simulink model "test_topo"  (R2023b)
settings: Solver=FixedStepAuto  StartTime=0  StopTime=0.1e-3  FixedStep=1e-9  RelTol=1e-3
values from neighbouring files (symbols this model uses):
  C = 34e-6    (= 3.4e-05)    [code_lsandtrain.m]
  It = 2310    [code_lsandtrain.m]
  L = 3.5e-6    (= 3.5e-06)    [code_lsandtrain.m]
  Lc = Lc*2    (= 8e-07)    [code_lsandtrain.m]
  Ld = 2.5e-7    (= 2.5e-07)    [code_lsandtrain.m]
  Lr = 3e-7    (= 3e-07)    [code_lsandtrain.m]
  R = 0.65    [code_lsandtrain.m]
  Ud = 2500    [code_lsandtrain.m]
undefined symbols (not defined in the file or in its folder): Udc
libraries: spsSeriesRLCBranchLib x47, spsVoltageMeasurementLib x38, spsDiodeLib x18, spsControlledCurrentSourceLib x9, spsCurrentMeasurementLib x9, spsDCVoltageSourceLib x9, spsIGBTDiodeLib x9, sps_lib x1
settings Model: Creator=Jhchen  LastModifiedBy=Jhchen
settings DataIOCC: ReturnWorkspaceOutputs=off

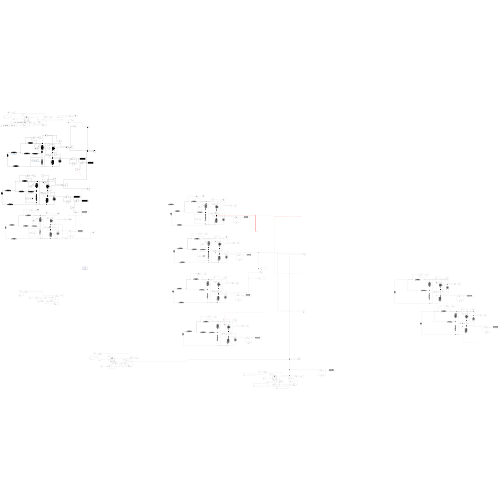
[thumbnail: Simulink's stored preview of the top-level diagram]
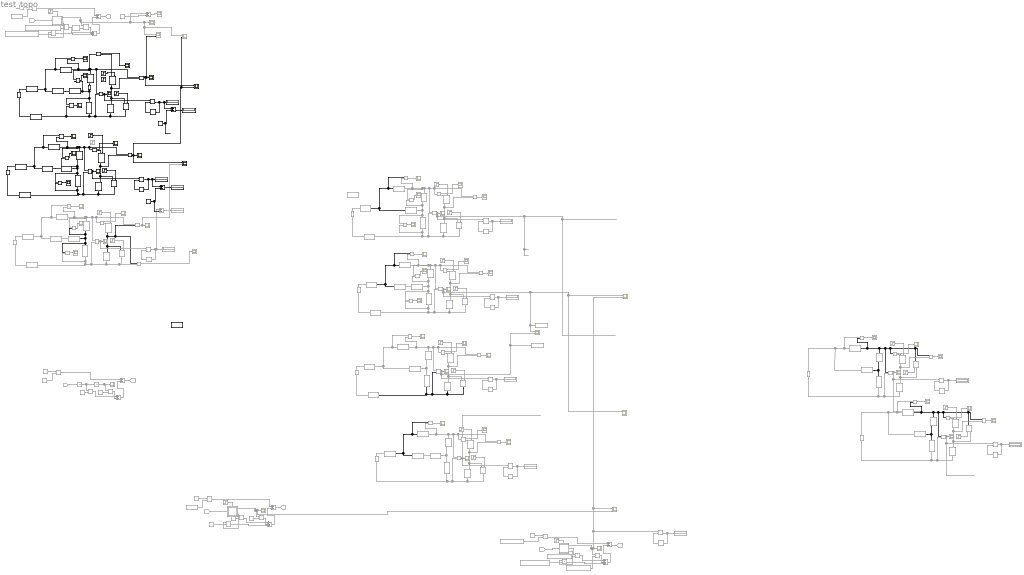
== system test_topo ==
  Add : Sum  Commented=on
  Add{1,3,5,7,10..11} (6 alike) : Sum  Commented=on  Inputs=+-
  Add2 : Sum  Commented=on  Inputs=+++
  Add4 : Sum  Commented=on  Inputs=+++
  Add6 : Sum  Inputs=+-
  Add8 : Sum  Inputs=+-
  Add9 : Sum  Commented=on  Inputs=+++
  Constant : Constant  Commented=on  Value=2400
  Constant1 : Constant  Commented=on  Value=L*C
  Constant10 : Constant  Commented=on  Value=R/(L*Lr*C+L*Lc*C+Lc*Lr*C)
  Constant11 : Constant  Commented=on  Value=R/(L*Lr*C+L*Lc*C+Lc*Lr*C)
  Constant12 : Constant  Commented=on  Value=(L+Lr)/(L*Lr*C+L*Lc*C+Lc*Lr*C)
  Constant13 : Constant  Commented=on  Value=(L*R*C+Lc*C*R)/(L*Lr*C+L*Lc*C+Lc*Lr*C)
  Constant14 : Constant  Value=Ud
  Constant15 : Constant  Value=Ud
  Constant16 : Constant  Commented=on  Value=Ud
  Constant17 : Constant  Commented=on  Value=(C*(L*Lc+Lc*Ld+Lc*Lr+Lr*L+Lr*Ld))/R
  Constant18 : Constant  Commented=on  Value=C*(L*Lc+Lc*Ld+Lc*Lr+Lr*L+Lr*Ld)/R
  Constant19 : Constant  Commented=on  Value=C*(L*Lc+Lc*Ld+Lc*Lr+Lr*L+Lr*Ld)/((L+Ld+Lr))
  Constant2 : Constant  Commented=on  Value=L*C
  Constant20 : Constant  Commented=on  Value=C*(L*Lc+Lc*Ld+Lc*Lr+Lr*L+Lr*Ld)/(C*R*(Lc+L+Ld))
  Constant21 : Constant  Commented=on  Value=Ud
  Constant3 : Constant  Commented=on  Value=R*C
  Constant4 : Constant  Commented=on  Value=Udc
  Constant5 : Constant  Commented=on  Value=L*C*Lc/R
  Constant6 : Constant  Commented=on  Value=L*C*Lc/R
  Constant7 : Constant  Commented=on  Value=Lc*C
  Constant8 : Constant  Commented=on  Value=L*Lc/R/(Lc+L)
  Constant9 : Constant  Commented=on  Value=Udc
  Controlled Current Source{1..7} (7 alike) : spsControlledCurrentSourceLib/Controlled Current Source  Commented=on  Initialize=on  Source_Type=AC  Amplitude=0  Phase=0  Frequency=0  Measurements=None
  Controlled Current Source8 : spsControlledCurrentSourceLib/Controlled Current Source  Initialize=on  Source_Type=AC  Amplitude=0  Phase=0  Frequency=0  Measurements=None
  Controlled Current Source9 : spsControlledCurrentSourceLib/Controlled Current Source  Initialize=on  Source_Type=AC  Amplitude=0  Phase=0  Frequency=0  Measurements=None
  Current Measurement{1..7} (7 alike) : spsCurrentMeasurementLib/Current Measurement  Commented=on  PhasorSimulation=off  OutputType=Complex  PSBequivalent=0
  Current Measurement8 : spsCurrentMeasurementLib/Current Measurement  PhasorSimulation=off  OutputType=Complex  PSBequivalent=0
  Current Measurement9 : spsCurrentMeasurementLib/Current Measurement  PhasorSimulation=off  OutputType=Complex  PSBequivalent=0
  DC Voltage Source1 : spsDCVoltageSourceLib/DC Voltage Source  Commented=on  Amplitude=Udc  Measurements=None
  DC Voltage Source2 : spsDCVoltageSourceLib/DC Voltage Source  Commented=on  Amplitude=2400  Measurements=None
  DC Voltage Source3 : spsDCVoltageSourceLib/DC Voltage Source  Commented=on  Amplitude=2400  Measurements=None
  DC Voltage Source4 : spsDCVoltageSourceLib/DC Voltage Source  Commented=on  Amplitude=2400  Measurements=None
  DC Voltage Source5 : spsDCVoltageSourceLib/DC Voltage Source  Commented=on  Amplitude=Udc  Measurements=None
  DC Voltage Source6 : spsDCVoltageSourceLib/DC Voltage Source  Commented=on  Amplitude=2500  Measurements=None
  DC Voltage Source7 : spsDCVoltageSourceLib/DC Voltage Source  Commented=on  Amplitude=Ud  Measurements=None
  DC Voltage Source8 : spsDCVoltageSourceLib/DC Voltage Source  Amplitude=Ud  Measurements=None
  DC Voltage Source9 : spsDCVoltageSourceLib/DC Voltage Source  Amplitude=Ud  Measurements=None
  Delay{1..8} (8 alike) : Delay  Commented=on  DelayLength=1
  Delay10 : Delay  DelayLength=1
  Delay9 : Delay  DelayLength=1
  Diode{1..14} (14 alike) : spsDiodeLib/Diode  Commented=on  Ron=0.001  Lon=0  Vf=0.8  IC=0  UseSnubber=0  Rs=500  Cs=250e-9  Measurements=on
  Diode{15..18} (4 alike) : spsDiodeLib/Diode  Ron=0.001  Lon=0  Vf=0.8  IC=0  UseSnubber=0  Rs=500  Cs=250e-9  Measurements=on
  Display{1..8,11} (9 alike) : Display  Commented=on
  Display{9..10,12..13} (4 alike) : Display
  Divide{,1..6,11..14} (11 alike) : Product  Commented=on  Inputs=*/
  Divide{7..10} (4 alike) : Product  Commented=on  Inputs=**
  From : From  Commented=on  GotoTag=vc2
  From1 : From  Commented=on  GotoTag=vc3
  From2 : From  Commented=on  GotoTag=vc4
  From3 : From  Commented=on  GotoTag=vc3
  Goto : Goto  Commented=on  GotoTag=vc2
  Goto1 : Goto  Commented=on  GotoTag=vc3
  Goto2 : Goto  Commented=on  GotoTag=vc4
  Goto3 : Goto  Commented=on  GotoTag=vc3
  IGBT/Diode{1..7} (7 alike) : spsIGBTDiodeLib/IGBT//Diode  Commented=on  Ron=0.39e-3  Rs=1e5  Cs=inf  Measurements=on
  IGBT/Diode8 : spsIGBTDiodeLib/IGBT//Diode  Ron=0.39e-3  Rs=1e5  Cs=inf  Measurements=on
  IGBT/Diode9 : spsIGBTDiodeLib/IGBT//Diode  Ron=0.39e-3  Rs=1e5  Cs=inf  Measurements=on
  Integrator1 : Integrator  Commented=on  InitialCondition=2400
  Integrator3 : Integrator  Commented=on  InitialCondition=1750/C
  Max{1..8} (8 alike) : MinMax  Commented=on  Function=max  Inputs=2
  Max10 : MinMax  Function=max  Inputs=2
  Max9 : MinMax  Function=max  Inputs=2
  Scope : Scope  NumInputPorts=2
  Scope{1..3,5..11,13..24,26..28,30..41,48,56,59} (40 alike) : Scope  Commented=on
  Scope12 : Scope  Commented=on  NumInputPorts=4
  Scope25 : Scope  Commented=on  NumInputPorts=3
  Scope{4,29,57..58} (4 alike) : Scope  Commented=on  NumInputPorts=2
  Scope{42..47,50..55} (12 alike) : Scope
  Scope49 : Scope  NumInputPorts=2
  Series RLC Branch{1,16,21,27} (4 alike) : spsSeriesRLCBranchLib/Series RLC Branch  Commented=on  LConnTagsString=__new0  RConnTagsString=__new0  BranchType=L  Resistance=0.00001  Inductance=L  SetiL0=off  InitialCurrent=4000  Capacitance=1e-6  Setx0=off  InitialVoltage=0  Measurements=None
  Series RLC Branch10 : spsSeriesRLCBranchLib/Series RLC Branch  Commented=on  LConnTagsString=__new0  RConnTagsString=__new0  BranchType=L  Resistance=1  Inductance=L  SetiL0=off  InitialCurrent=0  Capacitance=1e-6  Setx0=off  InitialVoltage=0  Measurements=None
  Series RLC Branch{4..6,11,24,34} (6 alike) : spsSeriesRLCBranchLib/Series RLC Branch  Commented=on  LConnTagsString=__new0  RConnTagsString=__new0  BranchType=R  Resistance=R  Inductance=1e-3  SetiL0=off  InitialCurrent=0  Capacitance=1e-6  Setx0=off  InitialVoltage=0  Measurements=None
  Series RLC Branch{7,9,12,14,17,30} (6 alike) : spsSeriesRLCBranchLib/Series RLC Branch  Commented=on  LConnTagsString=__new0  RConnTagsString=__new0  BranchType=C  Resistance=1  Inductance=1e-3  SetiL0=off  InitialCurrent=0  Capacitance=C  Setx0=off  InitialVoltage=0  Measurements=None
  Series RLC Branch13 : spsSeriesRLCBranchLib/Series RLC Branch  Commented=on  LConnTagsString=__new0  RConnTagsString=__new0  BranchType=L  Resistance=1  Inductance=L  SetiL0=off  InitialCurrent=0  Capacitance=1e-6  Setx0=off  InitialVoltage=0  Measurements=None
  Series RLC Branch15 : spsSeriesRLCBranchLib/Series RLC Branch  Commented=on  LConnTagsString=__new0  RConnTagsString=__new0  BranchType=L  Resistance=0.00001  Inductance=Lc/2  SetiL0=off  InitialCurrent=4000  Capacitance=1e-6  Setx0=off  InitialVoltage=0  Measurements=None
  Series RLC Branch18 : spsSeriesRLCBranchLib/Series RLC Branch  Commented=on  LConnTagsString=__new0  RConnTagsString=__new0  BranchType=L  Resistance=0.00001  Inductance=Lc  SetiL0=off  InitialCurrent=4000  Capacitance=1e-6  Setx0=off  InitialVoltage=0  Measurements=None
  Series RLC Branch19 : spsSeriesRLCBranchLib/Series RLC Branch  Commented=on  LConnTagsString=__new0  RConnTagsString=__new0  BranchType=L  Resistance=1  Inductance=Lc  SetiL0=off  InitialCurrent=4000  Capacitance=1e-6  Setx0=off  InitialVoltage=0  Measurements=None
  Series RLC Branch2 : spsSeriesRLCBranchLib/Series RLC Branch  Commented=on  LConnTagsString=__new0  RConnTagsString=__new0  BranchType=L  Resistance=1  Inductance=Lc/2  SetiL0=off  InitialCurrent=4000  Capacitance=1e-6  Setx0=off  InitialVoltage=0  Measurements=None
  Series RLC Branch{20,23,29,33} (4 alike) : spsSeriesRLCBranchLib/Series RLC Branch  Commented=on  LConnTagsString=__new0  RConnTagsString=__new0  BranchType=L  Resistance=1  Inductance=Lr  SetiL0=off  InitialCurrent=4000  Capacitance=1e-6  Setx0=off  InitialVoltage=0  Measurements=None
  Series RLC Branch22 : spsSeriesRLCBranchLib/Series RLC Branch  Commented=on  LConnTagsString=__new0  RConnTagsString=__new0  BranchType=L  Resistance=1  Inductance=Lc*2  SetiL0=off  InitialCurrent=4000  Capacitance=1e-6  Setx0=off  InitialVoltage=0  Measurements=None
  Series RLC Branch25 : spsSeriesRLCBranchLib/Series RLC Branch  Commented=on  LConnTagsString=__new0  RConnTagsString=__new0  BranchType=L  Resistance=0.00001  Inductance=2e-7  SetiL0=off  InitialCurrent=4000  Capacitance=1e-6  Setx0=off  InitialVoltage=0  Measurements=None
  Series RLC Branch26 : spsSeriesRLCBranchLib/Series RLC Branch  Commented=on  LConnTagsString=__new0  RConnTagsString=__new0  BranchType=L  Resistance=1  Inductance=2e-7  SetiL0=off  InitialCurrent=4000  Capacitance=1e-6  Setx0=off  InitialVoltage=0  Measurements=None
  Series RLC Branch28 : spsSeriesRLCBranchLib/Series RLC Branch  Commented=on  LConnTagsString=__new0  RConnTagsString=__new0  BranchType=R  Resistance=0.7172  Inductance=1e-3  SetiL0=off  InitialCurrent=0  Capacitance=1e-6  Setx0=off  InitialVoltage=0  Measurements=None
  Series RLC Branch3 : spsSeriesRLCBranchLib/Series RLC Branch  Commented=on  LConnTagsString=__new0  RConnTagsString=__new0  BranchType=L  Resistance=0.00001  Inductance=3.5e-6  SetiL0=off  InitialCurrent=4000  Capacitance=1e-6  Setx0=off  InitialVoltage=0  Measurements=None
  Series RLC Branch31 : spsSeriesRLCBranchLib/Series RLC Branch  Commented=on  LConnTagsString=__new0  RConnTagsString=__new0  BranchType=L  Resistance=0.00001  Inductance=Lc  SetiL0=off  InitialCurrent=4000  Capacitance=1e-6  Setx0=off  InitialVoltage=0  Measurements=None
  Series RLC Branch32 : spsSeriesRLCBranchLib/Series RLC Branch  Commented=on  LConnTagsString=__new0  RConnTagsString=__new0  BranchType=L  Resistance=1  Inductance=Lc  SetiL0=off  InitialCurrent=4000  Capacitance=1e-6  Setx0=off  InitialVoltage=0  Measurements=None
  Series RLC Branch35 : spsSeriesRLCBranchLib/Series RLC Branch  LConnTagsString=__new0  RConnTagsString=__new0  BranchType=L  Resistance=0.00001  Inductance=L  SetiL0=off  InitialCurrent=4000  Capacitance=1e-6  Setx0=off  InitialVoltage=0  Measurements=None
  Series RLC Branch36 : spsSeriesRLCBranchLib/Series RLC Branch  LConnTagsString=__new0  RConnTagsString=__new0  BranchType=C  Resistance=1  Inductance=1e-3  SetiL0=off  InitialCurrent=0  Capacitance=C  Setx0=off  InitialVoltage=0  Measurements=None
  Series RLC Branch37 : spsSeriesRLCBranchLib/Series RLC Branch  LConnTagsString=__new0  RConnTagsString=__new0  BranchType=L  Resistance=0.00001  Inductance=Lc/2  SetiL0=off  InitialCurrent=4000  Capacitance=1e-6  Setx0=off  InitialVoltage=0  Measurements=None
  Series RLC Branch38 : spsSeriesRLCBranchLib/Series RLC Branch  LConnTagsString=__new0  RConnTagsString=__new0  BranchType=L  Resistance=1  Inductance=Lc/2  SetiL0=off  InitialCurrent=4000  Capacitance=1e-6  Setx0=off  InitialVoltage=0  Measurements=None
  Series RLC Branch39 : spsSeriesRLCBranchLib/Series RLC Branch  LConnTagsString=__new0  RConnTagsString=__new0  BranchType=L  Resistance=0.00001  Inductance=L  SetiL0=off  InitialCurrent=4000  Capacitance=1e-6  Setx0=off  InitialVoltage=0  Measurements=None
  Series RLC Branch40 : spsSeriesRLCBranchLib/Series RLC Branch  LConnTagsString=__new0  RConnTagsString=__new0  BranchType=R  Resistance=R  Inductance=1e-3  SetiL0=off  InitialCurrent=0  Capacitance=1e-6  Setx0=off  InitialVoltage=0  Measurements=None
  Series RLC Branch41 : spsSeriesRLCBranchLib/Series RLC Branch  LConnTagsString=__new0  RConnTagsString=__new0  BranchType=C  Resistance=1  Inductance=1e-3  SetiL0=off  InitialCurrent=0  Capacitance=C  Setx0=off  InitialVoltage=0  Measurements=None
  Series RLC Branch42 : spsSeriesRLCBranchLib/Series RLC Branch  LConnTagsString=__new0  RConnTagsString=__new0  BranchType=L  Resistance=0.00001  Inductance=Lc/2  SetiL0=off  InitialCurrent=4000  Capacitance=1e-6  Setx0=off  InitialVoltage=0  Measurements=None
  Series RLC Branch43 : spsSeriesRLCBranchLib/Series RLC Branch  LConnTagsString=__new0  RConnTagsString=__new0  BranchType=L  Resistance=1  Inductance=Lc/2  SetiL0=off  InitialCurrent=4000  Capacitance=1e-6  Setx0=off  InitialVoltage=0  Measurements=None
  Series RLC Branch44 : spsSeriesRLCBranchLib/Series RLC Branch  LConnTagsString=__new0  RConnTagsString=__new0  BranchType=R  Resistance=R  Inductance=1e-3  SetiL0=off  InitialCurrent=0  Capacitance=1e-6  Setx0=off  InitialVoltage=0  Measurements=None
  Series RLC Branch45 : spsSeriesRLCBranchLib/Series RLC Branch  LConnTagsString=__new0  RConnTagsString=__new0  BranchType=L  Resistance=1  Inductance=Lr  SetiL0=off  InitialCurrent=4000  Capacitance=1e-6  Setx0=off  InitialVoltage=0  Measurements=None
  Series RLC Branch46 : spsSeriesRLCBranchLib/Series RLC Branch  LConnTagsString=__new0  RConnTagsString=__new0  BranchType=L  Resistance=1  Inductance=Ld  SetiL0=off  InitialCurrent=4000  Capacitance=1e-6  Setx0=off  InitialVoltage=0  Measurements=None
  Series RLC Branch47 : spsSeriesRLCBranchLib/Series RLC Branch  LConnTagsString=__new0  RConnTagsString=__new0  BranchType=L  Resistance=0.00001  Inductance=Lr  SetiL0=off  InitialCurrent=4000  Capacitance=1e-6  Setx0=off  InitialVoltage=0  Measurements=None
  Series RLC Branch8 : spsSeriesRLCBranchLib/Series RLC Branch  Commented=on  LConnTagsString=__new0  RConnTagsString=__new0  BranchType=C  Resistance=1  Inductance=1e-3  SetiL0=off  InitialCurrent=0  Capacitance=3.4e-5  Setx0=off  InitialVoltage=0  Measurements=None
  Step{1..2,8,14,16} (5 alike) : Step  Commented=on  Time=6e-5  Before=1  After=0  SampleTime=0
  Step10 : Step  Commented=on  Time=0  Before=It  After=It  SampleTime=0
  Step11 : Step  Commented=on  Time=6e-5  SampleTime=0
  Step12 : Step  Commented=on  Time=6e-5  SampleTime=0
  Step13 : Step  Commented=on  Time=0  Before=1750  After=1750  SampleTime=0
  Step15 : Step  Commented=on  Time=0  Before=It  After=It  SampleTime=0
  Step17 : Step  Time=0  Before=It  After=It  SampleTime=0
  Step18 : Step  Commented=on  Time=0  Before=1  After=0  SampleTime=0
  Step19 : Step  Time=0  Before=It  After=It  SampleTime=0
  Step20 : Step  Commented=on  Time=6e-5  SampleTime=0
  Step21 : Step  Time=0  Before=1  After=0  SampleTime=0
  Step22 : Step  Time=6e-5  Before=1  After=0  SampleTime=0
  Step23 : Step  Time=6e-5  Before=1  After=0  SampleTime=0
  Step3 : Step  Commented=on  Time=0  Before=It  After=It  SampleTime=0
  Step4 : Step  Commented=on  Time=0  Before=1  After=0  SampleTime=0
  Step5 : Step  Commented=on  Time=0  Before=1750  After=1750  SampleTime=0
  Step6 : Step  Commented=on  Time=0  Before=1  After=0  SampleTime=0
  Step7 : Step  Commented=on  Time=0  Before=1750  After=1750  SampleTime=0
  Step9 : Step  Commented=on  Time=0  Before=4000  After=4000  SampleTime=0
  Subsystem : Subsystem  Commented=on
  Subsystem1 : Subsystem  Commented=on
  Subsystem2 : Subsystem  Commented=on
  To Workspace : ToWorkspace  Commented=on  VariableName=lc  SaveFormat=Structure With Time  SampleTime=-1
  To Workspace1 : ToWorkspace  Commented=on  VariableName=lclr  SaveFormat=Structure With Time  SampleTime=-1
  Voltage Measurement{1..27,33} (28 alike) : spsVoltageMeasurementLib/Voltage Measurement  Commented=on  PhasorSimulation=off  OutputType=Complex  PSBequivalent=0
  Voltage Measurement{28..32,34..38} (10 alike) : spsVoltageMeasurementLib/Voltage Measurement  PhasorSimulation=off  OutputType=Complex  PSBequivalent=0
  powergui : sps_lib/powergui  Priority=1  SimulationMode=Discrete  SampleTime=1e-9  frequency=60  Iterations=50  frequencyindice=0  Pbase=100e6  ErrMax=1e-4  UnitsV=kV  UnitsW=MW  buscounter=0  FunctionMessages=off  echomessages=off  EnableUseOfTLC=off  CurrentSourceSwitches=off  DisableSnubberDevices=off  DisableRonSwitches=off  DisableVfSwitches=off  DisplayEquations=off  AutomaticDiscreteSolvers=off  SolverType=Tustin/Backward Euler (TBE)  Interpol=off  ExternalGateDelay=off  methode=off  Ts=100  x0status=blocks  SPID=on  SwTol=0  HookPort=off  NonlinearTolerance=1e-4  nMaxIteration=100  ContinueOnMaxIteration=off  RestoreLinks=warning  ResistiveCurrentMeasurement=off  Frange=[0:2:500]  Ylog=off  Xlog=on  ShowGrid=off  save=off  variable=ZData  structure=0  ZoomFFT=off  StartTime=0.0  cycles=1  DisplayStyle=1  fundamental=60  FreqAxis=off  MaxFrequency=1000  frequencyindicesteady=1  RmsSteady=1  display=off
  wires:
  Constant/1 -> Divide/1
  Constant1/1 -> Divide/2
  From/1 -> Integrator3/1
  Integrator3/1 -> Divide1/1, Integrator1/1
  Add/1 -> Add1/2
  Add1/1 -> Goto/1
  Constant3/1 -> Divide1/2
  Constant2/1 -> Divide2/2
  Integrator1/1 -> Scope5/1, Divide2/1
  Divide2/1 -> Add/2
  Divide/1 -> Add1/1
  Divide1/1 -> Add/1
  Divide4/1 -> Add2/1
  Divide3/1 -> Add3/1
  Divide5/1 -> Add2/2
  Constant6/1 -> Divide5/2
  Constant7/1 -> Divide4/2
  Add3/1 -> Goto1/1
  Add2/1 -> Add3/2
  Constant5/1 -> Divide3/2
  Constant4/1 -> Divide3/1
  Constant8/1 -> Divide6/2
  Divide6/1 -> Add2/3
  Divide10/1 -> Add4/3
  Constant13/1 -> Divide10/2
  Constant9/1 -> Divide7/1
  Constant10/1 -> Divide7/2
  Add4/1 -> Add5/2
  Add5/1 -> Goto2/1
  Constant12/1 -> Divide8/2
  Constant11/1 -> Divide9/2
  Divide9/1 -> Add4/2
  Divide7/1 -> Add5/1
  Divide8/1 -> Add4/1
  Voltage Measurement6/1 -> Max2/1, Scope14/1
  Voltage Measurement8/1 -> Scope16/1
  Voltage Measurement7/1 -> Scope15/1
  Step4/1 -> IGBT/Diode2/1
  Current Measurement2/1 -> Scope13/1
  Max2/1 -> Delay2/1, Display2/1
  Delay2/1 -> Max2/2
  Step5/1 -> Controlled Current Source2/1
  Voltage Measurement9/1 -> Max3/1, Scope18/1
  Voltage Measurement11/1 -> Scope20/1
  Voltage Measurement10/1 -> Scope19/1
  Step6/1 -> IGBT/Diode3/1
  Current Measurement3/1 -> Scope17/1
  Max3/1 -> Delay3/1, Display3/1
  Delay3/1 -> Max3/2
  Step7/1 -> Controlled Current Source3/1
  Step2/1 -> IGBT/Diode1/1
  Voltage Measurement3/1 -> Max1/1, Scope6/1
  Voltage Measurement4/1 -> Scope8/1
  Voltage Measurement5/1 -> Scope9/1
  Current Measurement1/1 -> Scope10/1
  Max1/1 -> Delay1/1, Display1/1
  Delay1/1 -> Max1/2
  Step9/1 -> Controlled Current Source1/1
  Step3/1 -> Controlled Current Source4/1
  Delay4/1 -> Max4/2
  Max4/1 -> Display4/1, Delay4/1
  Current Measurement4/1 -> Scope1/1
  Voltage Measurement12/1 -> Scope21/1
  Voltage Measurement2/1 -> Scope3/1
  Voltage Measurement1/1 -> Max4/1, Scope4/2, To Workspace1/1, Scope2/1
  Step1/1 -> IGBT/Diode4/1
  Step8/1 -> IGBT/Diode5/1
  Voltage Measurement13/1 -> To Workspace/1, Scope4/1, Scope29/1, Scope25/1, Max5/1, Scope23/1
  Voltage Measurement15/1 -> Scope26/1
  Voltage Measurement14/1 -> Scope24/1
  Current Measurement5/1 -> Scope22/1
  Max5/1 -> Delay5/1, Display5/1
  Delay5/1 -> Max5/2
  Step10/1 -> Controlled Current Source5/1
  Voltage Measurement16/1 -> Scope27/1
  Voltage Measurement17/1 -> Scope28/1
  Delay6/1 -> Max6/2
  Max6/1 -> Display6/1, Delay6/1
  Subsystem/1(Out1) -> Divide9/1, Max6/1, Scope29/2, Scope12/2, Scope11/1
  From2/1 -> Subsystem/1(In1)
  Subsystem/2(Out2) -> Divide8/1
  Subsystem/3(Out3) -> Divide10/1
  Step11/1 -> Subsystem/Enable
  Step12/1 -> Subsystem1/Enable
  Subsystem1/1(Out1) -> Divide5/1, Scope12/4, Scope7/1
  From1/1 -> Subsystem1/1(In1)
  Subsystem1/2(Out2) -> Divide4/1
  Subsystem1/3(Out3) -> Divide6/1
  Voltage Measurement22/1 -> Scope35/1
  Voltage Measurement21/1 -> Scope34/1
  Step13/1 -> Controlled Current Source6/1
  Delay7/1 -> Max7/2
  Max7/1 -> Display7/1, Delay7/1
  Current Measurement6/1 -> Scope30/1
  Voltage Measurement19/1 -> Scope32/1
  Voltage Measurement20/1 -> Scope33/1
  Voltage Measurement18/1 -> Scope31/1, Max7/1
  Step14/1 -> IGBT/Diode6/1
  Voltage Measurement26/1 -> Scope40/1
  Step16/1 -> IGBT/Diode7/1
  Voltage Measurement27/1 -> Scope41/1
  Voltage Measurement23/1 -> Max8/1, Scope37/1
  Current Measurement7/1 -> Scope36/1
  Max8/1 -> Delay8/1, Display8/1, Add7/1
  Voltage Measurement25/1 -> Scope39/1
  Voltage Measurement24/1 -> Scope/2, Scope38/1
  Delay8/1 -> Max8/2
  Step15/1 -> Controlled Current Source7/1
  Step17/1 -> Controlled Current Source8/1
  Delay9/1 -> Max9/2
  Voltage Measurement30/1 -> Scope45/1
  Max9/1 -> Add6/1, Display9/1, Delay9/1
  Current Measurement8/1 -> Scope42/1
  Voltage Measurement28/1 -> Scope43/1, Max9/1
  Voltage Measurement32/1 -> Scope47/1
  Step22/1 -> IGBT/Diode8/1
  Voltage Measurement31/1 -> Scope46/1
  Voltage Measurement33/1 -> Scope48/1
  Constant14/1 -> Add7/2, Add6/2
  Add7/1 -> Display11/1
  Add6/1 -> Display10/1
  Add8/1 -> Display12/1
  Constant15/1 -> Add8/2
  Voltage Measurement37/1 -> Scope54/1
  Voltage Measurement38/1 -> Scope55/1
  Voltage Measurement34/1 -> Max10/1, Scope51/1
  Current Measurement9/1 -> Scope50/1
  Max10/1 -> Delay10/1, Display13/1, Add8/1
  Voltage Measurement36/1 -> Scope53/1
  Delay10/1 -> Max10/2
  Step19/1 -> Controlled Current Source9/1
  Voltage Measurement29/1 -> Scope/1, Scope58/2, Scope49/2, Scope44/1
  Step23/1 -> IGBT/Diode9/1
  Voltage Measurement35/1 -> Scope49/1, Scope57/2, Scope52/1
  Step20/1 -> Subsystem2/Enable
  From3/1 -> Subsystem2/1(In1)
  Subsystem2/1(Out1) -> Divide13/1, Add11/1, Scope58/1, Scope57/1, Scope56/1
  Divide14/1 -> Add9/3
  Constant20/1 -> Divide14/2
  Divide12/1 -> Add9/1
  Constant17/1 -> Divide11/2
  Divide11/1 -> Add10/1
  Constant19/1 -> Divide12/2
  Add9/1 -> Add10/2
  Subsystem2/3(Out3) -> Divide14/1
  Add10/1 -> Goto3/1
  Subsystem2/2(Out2) -> Divide12/1
  Divide13/1 -> Add9/2
  Constant16/1 -> Divide11/1
  Constant18/1 -> Divide13/2
  Constant21/1 -> Add11/2
  Add11/1 -> Scope59/1
  connections:
  Diode4/RConn1 -- Series RLC Branch9/LConn1 -- Series RLC Branch5/RConn1
  Series RLC Branch10/RConn1 -- Voltage Measurement7/LConn2 -- Current Measurement2/LConn1 -- Voltage Measurement8/LConn1 -- Controlled Current Source2/RConn1 -- Voltage Measurement6/LConn1 -- Diode4/LConn1
  Voltage Measurement6/LConn2 -- Series RLC Branch9/RConn1 -- DC Voltage Source3/LConn1 -- Diode5/LConn1
  Voltage Measurement7/LConn1 -- DC Voltage Source3/RConn1 -- Series RLC Branch5/LConn1 -- Series RLC Branch10/LConn1
  Controlled Current Source2/LConn1 -- Diode5/RConn1 -- IGBT/Diode2/RConn1 -- Voltage Measurement8/LConn2
  Current Measurement2/RConn1 -- IGBT/Diode2/LConn1
  Diode6/RConn1 -- Series RLC Branch12/LConn1 -- Series RLC Branch11/RConn1
  Series RLC Branch13/RConn1 -- Voltage Measurement10/LConn2 -- Current Measurement3/LConn1 -- Voltage Measurement11/LConn1 -- Controlled Current Source3/RConn1 -- Voltage Measurement9/LConn1 -- Diode6/LConn1
  Voltage Measurement9/LConn2 -- Series RLC Branch12/RConn1 -- DC Voltage Source4/LConn1 -- Diode7/LConn1
  Voltage Measurement10/LConn1 -- DC Voltage Source4/RConn1 -- Series RLC Branch11/LConn1 -- Series RLC Branch13/LConn1
  Controlled Current Source3/LConn1 -- Diode7/RConn1 -- IGBT/Diode3/RConn1 -- Voltage Measurement11/LConn2
  Current Measurement3/RConn1 -- IGBT/Diode3/LConn1
  Current Measurement1/LConn1 -- Diode2/LConn1 -- Voltage Measurement4/LConn2 -- Series RLC Branch21/RConn1 -- Voltage Measurement3/LConn1 -- Voltage Measurement5/LConn1
  Series RLC Branch22/RConn1 -- Series RLC Branch21/LConn1 -- Voltage Measurement4/LConn1 -- Series RLC Branch23/LConn1
  Series RLC Branch7/LConn1 -- Series RLC Branch6/RConn1 -- Diode2/RConn1
  Diode3/RConn1 -- Voltage Measurement5/LConn2 -- IGBT/Diode1/RConn1 -- Controlled Current Source1/LConn1
  DC Voltage Source2/RConn1 -- Series RLC Branch22/LConn1
  Series RLC Branch6/LConn1 -- Series RLC Branch23/RConn1
  Current Measurement1/RConn1 -- IGBT/Diode1/LConn1
  Diode3/LConn1 -- DC Voltage Source2/LConn1 -- Series RLC Branch7/RConn1 -- Voltage Measurement3/LConn2 -- Controlled Current Source1/RConn1
  Voltage Measurement2/LConn2 -- Current Measurement4/LConn1 -- Voltage Measurement12/LConn1 -- Voltage Measurement1/LConn1 -- Diode1/LConn1 -- Series RLC Branch1/RConn1
  Series RLC Branch4/RConn1 -- Series RLC Branch14/LConn1 -- Diode1/RConn1
  Voltage Measurement12/LConn2 -- Diode8/RConn1 -- Controlled Current Source4/LConn1 -- IGBT/Diode4/RConn1
  Series RLC Branch14/RConn1 -- Diode8/LConn1 -- Controlled Current Source4/RConn1 -- Voltage Measurement1/LConn2 -- Series RLC Branch15/RConn1
  Series RLC Branch15/LConn1 -- DC Voltage Source1/LConn1
  Current Measurement4/RConn1 -- IGBT/Diode4/LConn1
  DC Voltage Source1/RConn1 -- Series RLC Branch2/LConn1
  Series RLC Branch1/LConn1 -- Series RLC Branch4/LConn1 -- Series RLC Branch2/RConn1 -- Voltage Measurement2/LConn1
  Current Measurement5/LConn1 -- Voltage Measurement14/LConn1 -- Voltage Measurement17/LConn1 -- Voltage Measurement15/LConn2 -- Series RLC Branch16/RConn1 -- Diode9/LConn1 -- Voltage Measurement13/LConn1
  Series RLC Branch19/RConn1 -- Series RLC Branch16/LConn1 -- Voltage Measurement15/LConn1 -- Series RLC Branch20/LConn1
  Series RLC Branch17/LConn1 -- Series RLC Branch24/RConn1 -- Voltage Measurement17/LConn2 -- Diode9/RConn1 -- Voltage Measurement16/LConn1
  Diode10/RConn1 -- Voltage Measurement14/LConn2 -- IGBT/Diode5/RConn1 -- Controlled Current Source5/LConn1
  Diode10/LConn1 -- Voltage Measurement16/LConn2 -- Series RLC Branch17/RConn1 -- Series RLC Branch18/RConn1 -- Voltage Measurement13/LConn2 -- Controlled Current Source5/RConn1
  Series RLC Branch24/LConn1 -- Series RLC Branch20/RConn1
  Current Measurement5/RConn1 -- IGBT/Diode5/LConn1
  DC Voltage Source5/RConn1 -- Series RLC Branch19/LConn1
  Series RLC Branch18/LConn1 -- DC Voltage Source5/LConn1
  Current Measurement6/LConn1 -- Voltage Measurement18/LConn1 -- Diode12/LConn1 -- Series RLC Branch3/RConn1 -- Voltage Measurement20/LConn2 -- Voltage Measurement22/LConn1 -- Voltage Measurement19/LConn1
  Series RLC Branch8/LConn1 -- Voltage Measurement21/LConn1 -- Diode12/RConn1 -- Voltage Measurement22/LConn2 -- Series RLC Branch28/RConn1
  Diode11/RConn1 -- Controlled Current Source6/LConn1 -- IGBT/Diode6/RConn1 -- Voltage Measurement19/LConn2
  Diode11/LConn1 -- Controlled Current Source6/RConn1 -- Voltage Measurement18/LConn2 -- Series RLC Branch25/RConn1 -- Series RLC Branch8/RConn1 -- Voltage Measurement21/LConn2
  Series RLC Branch25/LConn1 -- DC Voltage Source6/LConn1
  Series RLC Branch26/RConn1 -- Series RLC Branch28/LConn1 -- Voltage Measurement20/LConn1 -- Series RLC Branch3/LConn1
  Current Measurement6/RConn1 -- IGBT/Diode6/LConn1
  DC Voltage Source6/RConn1 -- Series RLC Branch26/LConn1
  Controlled Current Source7/RConn1 -- Voltage Measurement33/LConn2 -- Diode13/LConn1 -- Voltage Measurement26/LConn2 -- Series RLC Branch30/RConn1 -- Series RLC Branch31/RConn1 -- Voltage Measurement23/LConn2
  Diode14/RConn1 -- Voltage Measurement27/LConn2 -- Series RLC Branch30/LConn1 -- Voltage Measurement26/LConn1 -- Series RLC Branch34/RConn1
  Voltage Measurement25/LConn1 -- Series RLC Branch27/LConn1 -- Series RLC Branch33/LConn1 -- Series RLC Branch32/RConn1
  IGBT/Diode7/RConn1 -- Voltage Measurement33/LConn1 -- Voltage Measurement24/LConn2 -- Diode13/RConn1 -- Controlled Current Source7/LConn1
  Voltage Measurement23/LConn1 -- Voltage Measurement27/LConn1 -- Voltage Measurement25/LConn2 -- Series RLC Branch27/RConn1 -- Diode14/LConn1 -- Current Measurement7/LConn1 -- Voltage Measurement24/LConn1
  Series RLC Branch31/LConn1 -- DC Voltage Source7/LConn1
  DC Voltage Source7/RConn1 -- Series RLC Branch32/LConn1
  Current Measurement7/RConn1 -- IGBT/Diode7/LConn1
  Series RLC Branch34/LConn1 -- Series RLC Branch33/RConn1
  Voltage Measurement31/LConn2 -- Controlled Current Source8/RConn1 -- Diode15/LConn1 -- Voltage Measurement28/LConn2 -- Series RLC Branch37/RConn1 -- Series RLC Branch36/RConn1
  Voltage Measurement32/LConn2 -- Diode16/RConn1 -- Series RLC Branch40/RConn1 -- Voltage Measurement31/LConn1 -- Series RLC Branch36/LConn1
  Diode15/RConn1 -- IGBT/Diode8/RConn1 -- Voltage Measurement29/LConn2 -- Controlled Current Source8/LConn1
  Voltage Measurement30/LConn2 -- Voltage Measurement29/LConn1 -- Current Measurement8/LConn1 -- Voltage Measurement28/LConn1 -- Diode16/LConn1 -- Voltage Measurement32/LConn1 -- Series RLC Branch35/RConn1
  Current Measurement8/RConn1 -- IGBT/Diode8/LConn1
  DC Voltage Source8/RConn1 -- Series RLC Branch38/LConn1
  Series RLC Branch37/LConn1 -- DC Voltage Source8/LConn1
  Series RLC Branch38/RConn1 -- Series RLC Branch47/LConn1 -- Voltage Measurement30/LConn1 -- Series RLC Branch35/LConn1
  Voltage Measurement37/LConn2 -- Controlled Current Source9/RConn1 -- Diode17/LConn1 -- Voltage Measurement34/LConn2 -- Series RLC Branch41/RConn1 -- Series RLC Branch42/RConn1
  Diode17/RConn1 -- Controlled Current Source9/LConn1 -- Voltage Measurement35/LConn2 -- IGBT/Diode9/RConn1
  Voltage Measurement36/LConn2 -- Series RLC Branch39/RConn1 -- Voltage Measurement38/LConn1 -- Voltage Measurement35/LConn1 -- Voltage Measurement34/LConn1 -- Diode18/LConn1 -- Current Measurement9/LConn1
  Series RLC Branch45/RConn1 -- Series RLC Branch44/LConn1
  Series RLC Branch42/LConn1 -- DC Voltage Source9/LConn1
  DC Voltage Source9/RConn1 -- Series RLC Branch43/LConn1
  Voltage Measurement36/LConn1 -- Series RLC Branch39/LConn1 -- Series RLC Branch45/LConn1 -- Series RLC Branch43/RConn1
  Diode18/RConn1 -- Series RLC Branch46/LConn1
  Current Measurement9/RConn1 -- IGBT/Diode9/LConn1
  Voltage Measurement38/LConn2 -- Series RLC Branch46/RConn1 -- Series RLC Branch41/LConn1 -- Voltage Measurement37/LConn1 -- Series RLC Branch44/RConn1
  Series RLC Branch47/RConn1 -- Series RLC Branch40/LConn1

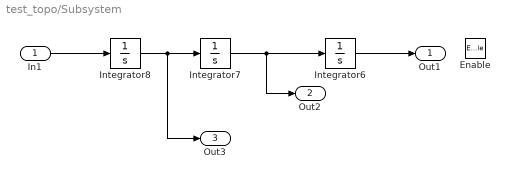
== system test_topo/Subsystem ==
  In1 : Inport
  Enable : EnablePort
  Integrator6 : Integrator  InitialCondition=Udc
  Integrator7 : Integrator  InitialCondition=It/C
  Integrator8 : Integrator
  Out1 : Outport
  Out2 : Outport  Port=2
  Out3 : Outport  Port=3
  wires:
  Integrator7/1 -> Out2/1, Integrator6/1
  Integrator8/1 -> Out3/1, Integrator7/1
  In1/1 -> Integrator8/1
  Integrator6/1 -> Out1/1

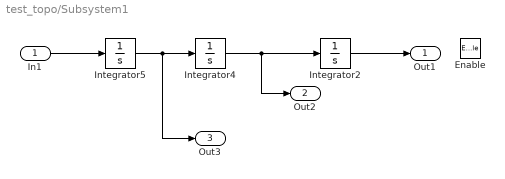
== system test_topo/Subsystem1 ==
  In1 : Inport
  Enable : EnablePort
  Integrator2 : Integrator  InitialCondition=Udc
  Integrator4 : Integrator  InitialCondition=It/C
  Integrator5 : Integrator
  Out1 : Outport
  Out2 : Outport  Port=2
  Out3 : Outport  Port=3
  wires:
  Integrator5/1 -> Out3/1, Integrator4/1
  Integrator4/1 -> Out2/1, Integrator2/1
  In1/1 -> Integrator5/1
  Integrator2/1 -> Out1/1

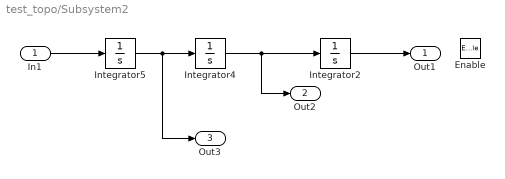
== system test_topo/Subsystem2 ==
  In1 : Inport
  Enable : EnablePort
  Integrator2 : Integrator  InitialCondition=Ud
  Integrator4 : Integrator  InitialCondition=It/C
  Integrator5 : Integrator
  Out1 : Outport
  Out2 : Outport  Port=2
  Out3 : Outport  Port=3
  wires:
  Integrator5/1 -> Out3/1, Integrator4/1
  Integrator4/1 -> Out2/1, Integrator2/1
  In1/1 -> Integrator5/1
  Integrator2/1 -> Out1/1
